simulink model "ModulacionFM"  (R2017b)
settings: Solver=VariableStepAuto  StartTime=0.0  StopTime=0.2  RelTol=1e-3
values from neighbouring files (symbols this model uses):
  f_delta = 50    [PracticaFMAgustinAvila.m]
  wc = 2000+wc_asignada    (= 2725)    [PracticaFMAgustinAvila.m]
libraries: powerlib_meascontrol x1, dspsrcs4 x1, simulink x1
settings Model: Creator=leand  LastModifiedBy=Agustin

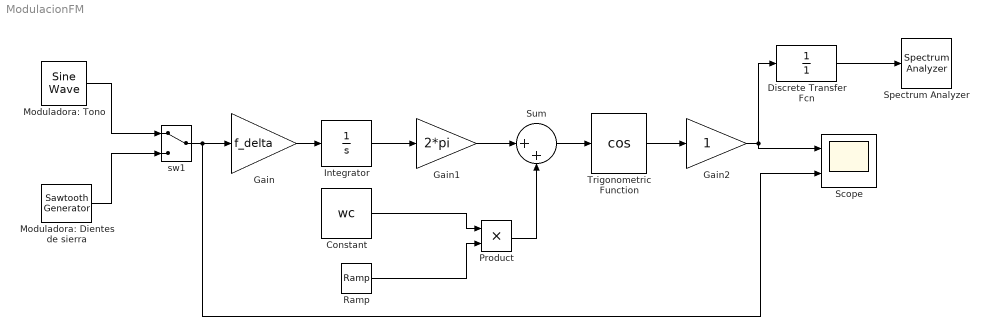
== system ModulacionFM ==
  Constant : Constant  Value=wc
  Discrete Transfer Fcn : DiscreteTransferFcn  Denominator=[1]
  Gain : Gain  Gain=f_delta
  Gain1 : Gain  Gain=2*pi
  Gain2 : Gain
  Integrator : Integrator
  Moduladora: Dientes de sierra : powerlib_meascontrol/Pulse & Signal Generators/Sawtooth Generator  Freq=10  Phase=180  Ts=1/10000
      settings: SourceProductName=Simscape Power Systems
  Moduladora: Tono : dspsrcs4/Sine Wave  Amplitude=1  Frequency=300  Phase=0  SampleMode=Discrete  OutComplex=Real  CompMethod=Trigonometric fcn  TableSize=Speed  SampleTime=1/10000  SamplesPerFrame=1  ResetState=Restart at time zero  OutputFrames=off  dataType=double  wordLen=16  udDataType=sfix(16)  fracBitsMode=Best precision  numFracBits=15  OutDataTypeStr=double  LastOutDataTypeStr=double
  Product : Product
  Ramp : simulink/Sources/Ramp  slope=1  start=0  X0=0
  Scope : Scope  NumInputPorts=2
  Spectrum Analyzer : SpectrumAnalyzer
  Sum : Sum  Inputs=|++
  Trigonometric Function : Trigonometry  Operator=cos  OutputSignalType=real
  sw1 : ManualSwitch
  wires:
  Moduladora: Tono/1 -> sw1/1
  Moduladora: Dientes de sierra/1 -> sw1/2
  Sum/1 -> Trigonometric Function/1
  Integrator/1 -> Gain1/1
  Constant/1 -> Product/1
  Ramp/1 -> Product/2
  Product/1 -> Sum/2
  Trigonometric Function/1 -> Gain2/1
  Gain/1 -> Integrator/1
  Gain2/1 -> Scope/1, Discrete Transfer Fcn/1
  Gain1/1 -> Sum/1
  Discrete Transfer Fcn/1 -> Spectrum Analyzer/1
  sw1/1 -> Scope/2, Gain/1
